simulink model "test_integrator_with_state_boundaries"  (R2014b)
settings: Solver=ode3  SolverMode=SingleTasking  StartTime=0.0  StopTime=Tsim  FixedStep=Ts  RelTol=1e-3
InitFcn:
  | config
libraries: simulink x1
settings Model: CovMetricSettings=dwe  CovHtmlReporting=off  covSaveCumulativeToWorkspaceVar=off  CovSaveSingleToWorkspaceVar=off  CovExternalEMLEnable=on  CovSFcnEnable=on  Creator=mnade  LastModifiedBy=nina
settings DataIOCC: LimitDataPoints=off  SaveFormat=StructureWithTime
settings DebuggingCC: SolverPrmCheckMsg=none  FrameProcessingCompatibilityMsg=error  SFUnexpectedBacktrackingDiag=error  SFNoUnconditionalDefaultTransitionDiag=error
settings HardwareCC: ProdBitPerPointer=64  ProdLargestAtomicFloat=Float  ProdIntDivRoundTo=Zero  ProdEndianess=LittleEndian  ProdHWDeviceType=Specified
settings ModelReferenceCC: PropagateSignalLabelsOutOfModel=on
settings GRTTargetCC: TargetLangStandard=C99 (ISO)  GeneratePreprocessorConditionals=Use local settings

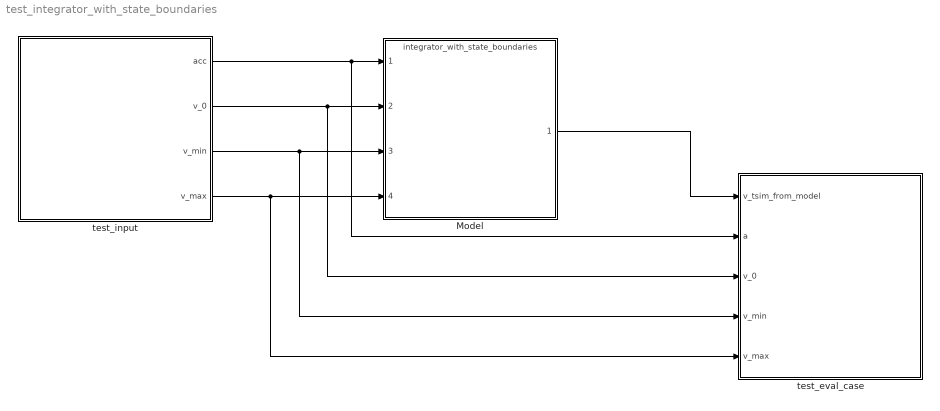
== system test_integrator_with_state_boundaries ==
  Model : ModelReference  ModelNameDialog=integrator_with_state_boundaries.slx  SimulationMode=Normal  ModelReferenceVersion=1.17  CopyOfModelName=integrator_with_state_boundaries.slx  DefaultDataLogging=on
  test_eval_case : Subsystem
  test_input : Subsystem
  wires:
  Model/1 -> test_eval_case/1(v_tsim_from_model)
  test_input/2(v_0) -> test_eval_case/3(v_0), Model/2
  test_input/3(v_min) -> test_eval_case/4(v_min), Model/3
  test_input/4(v_max) -> test_eval_case/5(v_max), Model/4
  test_input/1(acc) -> test_eval_case/2(a), Model/1

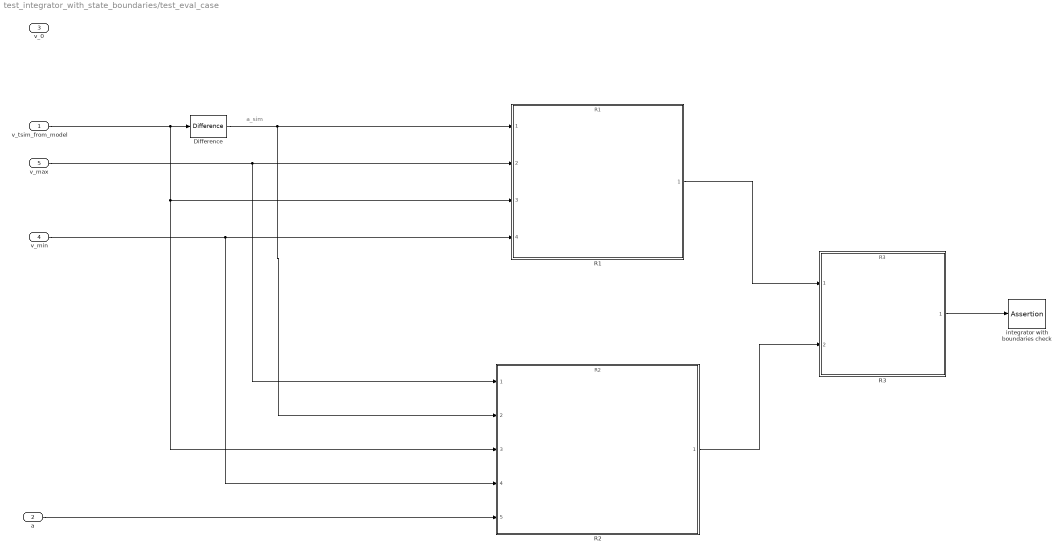
== system test_integrator_with_state_boundaries/test_eval_case ==
  note: a_sim
  v_tsim_from_model : Inport
  a : Inport  Port=2
  v_0 : Inport  Port=3
  v_min : Inport  Port=4
  v_max : Inport  Port=5
  Difference : simulink/Discrete/Difference  ICPrevInput=0.0  InputProcessing=Inherited  OutMin=[]  OutMax=[]  OutDataType=fixdt(1, 16)  OutScaling=2^-10  DoSatur=off
  R1 : ModelReference  ModelNameDialog=R1.slx  SimulationMode=Normal  ModelReferenceVersion=1.6  CopyOfModelName=R1.slx  DefaultDataLogging=on
  R2 : ModelReference  ModelNameDialog=R2.slx  SimulationMode=Normal  ModelReferenceVersion=1.5  CopyOfModelName=R2.slx  DefaultDataLogging=on
  R3 : ModelReference  ModelNameDialog=R3.slx  SimulationMode=Normal  ModelReferenceVersion=1.6  CopyOfModelName=R3.slx  DefaultDataLogging=on
  integrator with boundaries check : Assertion
  wires:
  v_tsim_from_model/1 -> R2/3, R1/3, Difference/1
  v_max/1 -> R2/1, R1/2
  v_min/1 -> R2/4, R1/4
  a/1 -> R2/5
  Difference/1 -> R2/2, R1/1
  R3/1 -> integrator with boundaries check/1
  R1/1 -> R3/1
  R2/1 -> R3/2

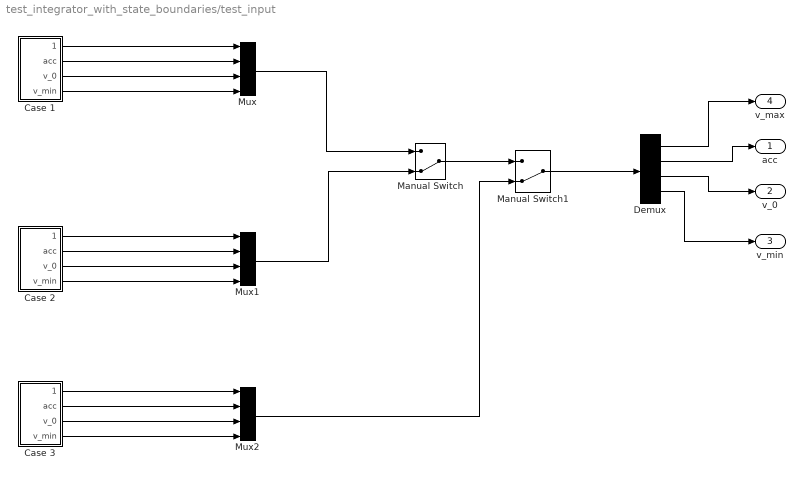
== system test_integrator_with_state_boundaries/test_input ==
  Case 1 : Subsystem
  Case 2 : Subsystem
  Case 3 : Subsystem
  Demux : Demux
  Manual Switch : ManualSwitch  CurrentSetting=0
  Manual Switch1 : ManualSwitch  CurrentSetting=0
  Mux : Mux
  Mux1 : Mux
  Mux2 : Mux
  acc : Outport
  v_0 : Outport  Port=2
  v_min : Outport  Port=3
  v_max : Outport  Port=4
  wires:
  Case 1/1(v_max) -> Mux/1
  Case 1/2(acc) -> Mux/2
  Case 1/3(v_0) -> Mux/3
  Case 1/4(v_min) -> Mux/4
  Case 2/1(v_max) -> Mux1/1
  Case 2/2(acc) -> Mux1/2
  Case 2/3(v_0) -> Mux1/3
  Case 2/4(v_min) -> Mux1/4
  Case 3/1(v_max) -> Mux2/1
  Case 3/2(acc) -> Mux2/2
  Case 3/3(v_0) -> Mux2/3
  Case 3/4(v_min) -> Mux2/4
  Demux/1 -> v_max/1
  Demux/2 -> acc/1
  Demux/3 -> v_0/1
  Demux/4 -> v_min/1
  Manual Switch1/1 -> Demux/1
  Mux/1 -> Manual Switch/1
  Mux1/1 -> Manual Switch/2
  Mux2/1 -> Manual Switch1/2
  Manual Switch/1 -> Manual Switch1/1

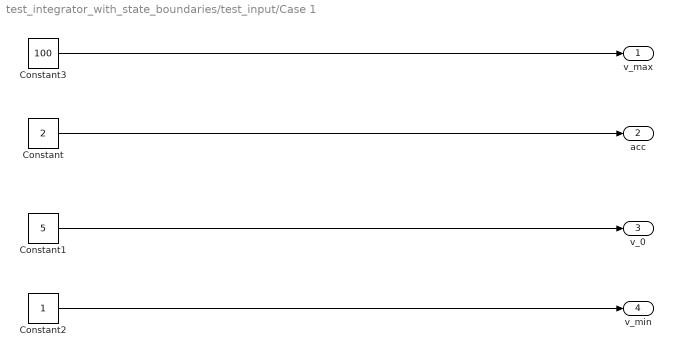
== system test_integrator_with_state_boundaries/test_input/Case 1 ==
  Constant : Constant  Value=2
  Constant1 : Constant  Value=5
  Constant2 : Constant
  Constant3 : Constant  Value=100
  v_max : Outport
  acc : Outport  Port=2
  v_0 : Outport  Port=3
  v_min : Outport  Port=4
  wires:
  Constant3/1 -> v_max/1
  Constant/1 -> acc/1
  Constant2/1 -> v_min/1
  Constant1/1 -> v_0/1

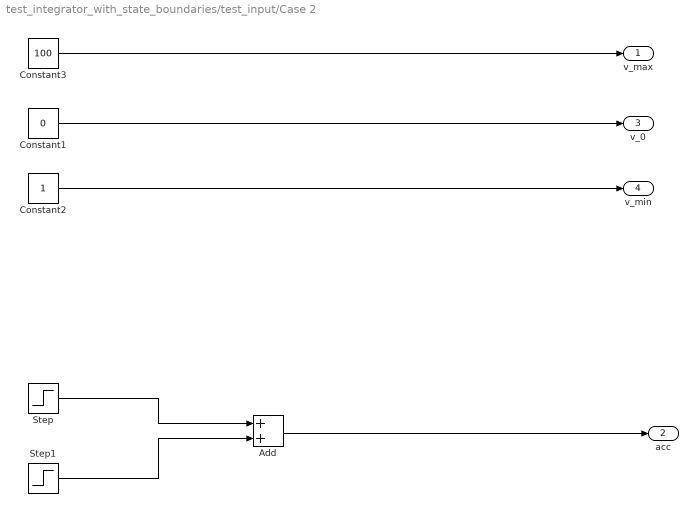
== system test_integrator_with_state_boundaries/test_input/Case 2 ==
  Add : Sum
  Constant1 : Constant  Value=0
  Constant2 : Constant
  Constant3 : Constant  Value=100
  Step : Step  After=2  SampleTime=0
  Step1 : Step  Time=60  After=-4  SampleTime=0
  v_max : Outport
  acc : Outport  Port=2
  v_0 : Outport  Port=3
  v_min : Outport  Port=4
  wires:
  Constant3/1 -> v_max/1
  Constant2/1 -> v_min/1
  Constant1/1 -> v_0/1
  Step/1 -> Add/1
  Step1/1 -> Add/2
  Add/1 -> acc/1

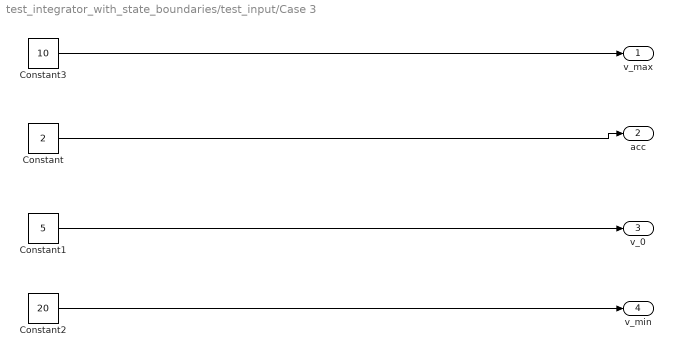
== system test_integrator_with_state_boundaries/test_input/Case 3 ==
  Constant : Constant  Value=2
  Constant1 : Constant  Value=5
  Constant2 : Constant  Value=20
  Constant3 : Constant  Value=10
  v_max : Outport
  acc : Outport  Port=2
  v_0 : Outport  Port=3
  v_min : Outport  Port=4
  wires:
  Constant3/1 -> v_max/1
  Constant/1 -> acc/1
  Constant2/1 -> v_min/1
  Constant1/1 -> v_0/1
